simulink model "doc_mer_and_evm"  (R2014a)
settings: Solver=VariableStepDiscrete  SolverMode=SingleTasking  StartTime=0.0  StopTime=10  RelTol=1e-3
PostLoadFcn:
  | qamRefConst = [-3.00000000000000 + 3.00000000000000i
  | -3.00000000000000 + 1.00000000000000i
  | -3.00000000000000 - 1.00000000000000i
  | -3.00000000000000 - 3.00000000000000i
  | -1.00000000000000 + 3.00000000000000i
  | -1.00000000000000 + 1.00000000000000i
  | -1.00000000000000 - 1.00000000000000i
  | -1.00000000000000 - 3.00000000000000i
  | 1.00000000000000 + 3.00000000000000i
  | 1.00000000000000 + 1.00000000000000i
  | 1.00000000000000 - 1.00000000000000i
  | 1.00000000000000 - 3.00000000000000i
  | 3.00000000000000 + 3.00000000000000i
  | 3.00000000000000 + 1.00000000000000i
  | 3.00000000000000 - 1.00000000000000i
  | 3.00000000000000 - 3.00000000000000i];
libraries: commutil2 x2, commrflib2 x1, commrandsrc2 x1, commdigbbndam3 x1
settings Model: Creator=The MathWorks Inc.
settings DataIOCC: SaveOutput=off  SaveTime=off
settings OptimizationCC: BooleanDataType=off  InlineParams=on  LocalBlockOutputs=off
settings DebuggingCC: AlgebraicLoopMsg=error  SingleTaskRateTransMsg=error

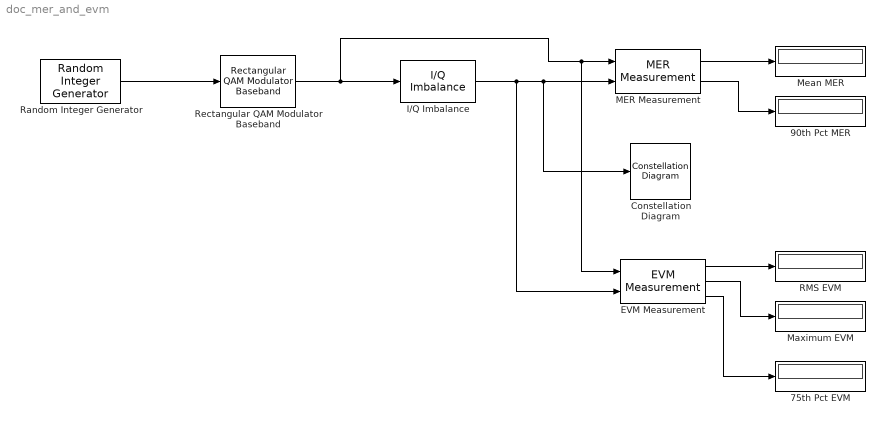
== system doc_mer_and_evm ==
  75th Pct EVM : Display
  90th Pct MER : Display
  Constellation Diagram : ConstellationDiagram
  EVM Measurement : commutil2/EVM Measurement  normMethod=Average reference signal power  averagePower=1  peakPower=1  maxOrMinOut=on  percentileOut=on  percentileVal=75  nSym=off
  I/Q Imbalance : commrflib2/I//Q Imbalance  ampImbal=1  phsImbal=15  Idc=0  Qdc=0
  MER Measurement : commutil2/MER Measurement  maxOrMinOut=off  percentileOut=on  percentileVal=90  nSym=off
  Maximum EVM : Display
  Mean MER : Display
  RMS EVM : Display
  Random Integer Generator : commrandsrc2/Random Integer Generator  mul=16  seed=37  Ts=0.001  frameBased=on  sampPerFrame=1000  orient=off  outDataType=double
  Rectangular QAM Modulator Baseband : commdigbbndam3/Rectangular QAM Modulator Baseband  M=16  InType=Integer  Enc=Gray  Mapping=[0:15]  PowType=Min. distance between symbols  MinDist=2  AvgPow=1  PeakPow=1  Ph=0  outDtype=double  outWordLen=16  outUDDataType=sfix(16)  outFracLenMode=Best precision  outFracLen=15
  wires:
  Random Integer Generator/1 -> Rectangular QAM Modulator Baseband/1
  Rectangular QAM Modulator Baseband/1 -> I/Q Imbalance/1, EVM Measurement/1, MER Measurement/1
  I/Q Imbalance/1 -> EVM Measurement/2, Constellation Diagram/1, MER Measurement/2
  MER Measurement/1 -> Mean MER/1
  MER Measurement/2 -> 90th Pct MER/1
  EVM Measurement/1 -> RMS EVM/1
  EVM Measurement/2 -> Maximum EVM/1
  EVM Measurement/3 -> 75th Pct EVM/1
